simulink model "P2"  (R2023b)
settings: Solver=VariableStepAuto  StartTime=0.0  StopTime=300  RelTol=1e-3
settings Model: Creator=ricar  LastModifiedBy=ricar

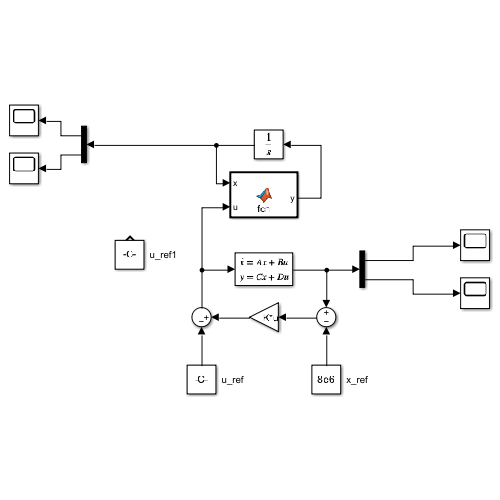
[thumbnail: Simulink's stored preview of the top-level diagram]
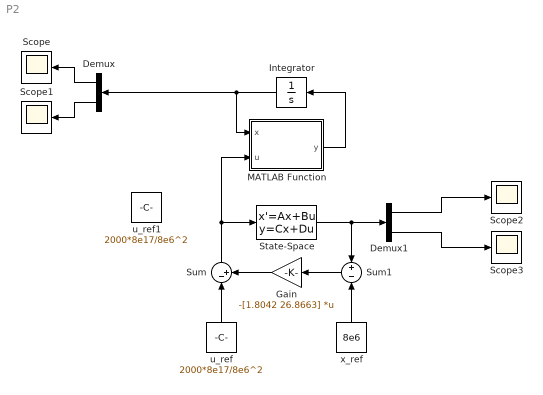
== system P2 ==
  Demux : Demux  Outputs=2
  Demux1 : Demux  Outputs=2
  Gain : Gain  Gain=-[1.8042 26.8663]  Multiplication=Matrix(K*u)
  Integrator : Integrator  InitialCondition=[8e6; 0]
  MATLAB Function : MATLAB Function  TreatAsAtomicUnit=on
  Scope{,1..3} (4 alike) : Scope
  State-Space : StateSpace  A=[0 1; 2*8e17/8e6^3 0]  B=[0;1/2000]  C=eye(2)  D=[0;0]  InitialCondition=[8e6, 0]  AllowTunableDMatrix=on
  Sum : Sum  Inputs=|-+
  Sum1 : Sum  Inputs=+|-
  u_ref : Constant  Value=2000*8e17/8e6^2
  u_ref1 : Constant  Value=2000*8e17/8e6^2
  x_ref : Constant  Value=8e6
  wires:
  MATLAB Function/1(y) -> Integrator/1
  Integrator/1 -> Demux/1, MATLAB Function/1(x)
  Demux/1 -> Scope/1
  Demux/2 -> Scope1/1
  State-Space/1 -> Sum1/1, Demux1/1
  Demux1/2 -> Scope3/1
  Demux1/1 -> Scope2/1
  Gain/1 -> Sum/2
  Sum/1 -> MATLAB Function/2(u), State-Space/1
  u_ref/1 -> Sum/1
  Sum1/1 -> Gain/1
  x_ref/1 -> Sum1/2

== matlab function P2/MATLAB Function ==
  data: x input; u input; y output
function y = fcn(x,u)

if x(1) <= 6378e3
    dx = [0;0];
else
dx = [x(2);-8e17/(x(1))^2+u/2000];
end


y = dx;
